simulink model "sininput"  (Simulink 4.00)
settings: Solver=ode45  StartTime=0.0  StopTime=10.0  RelTol=1e-3
settings Model: LastModifiedBy=administrator

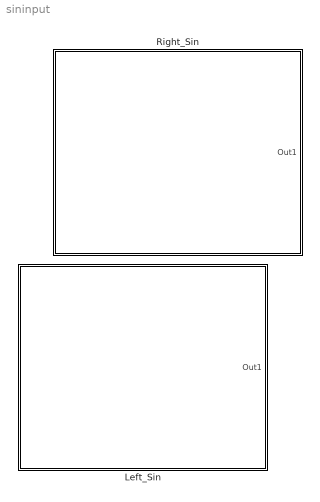
== system sininput ==
  Left_Sin : Subsystem
      settings: RTWFcnNameOpts=Auto  RTWFileNameOpts=Auto
      mask Display: disp('Left_Sin Roadspectrum')
  Right_Sin : Subsystem
      settings: RTWFcnNameOpts=Auto  RTWFileNameOpts=Auto
      mask Display: disp('Right_Sin Roadspectrum')

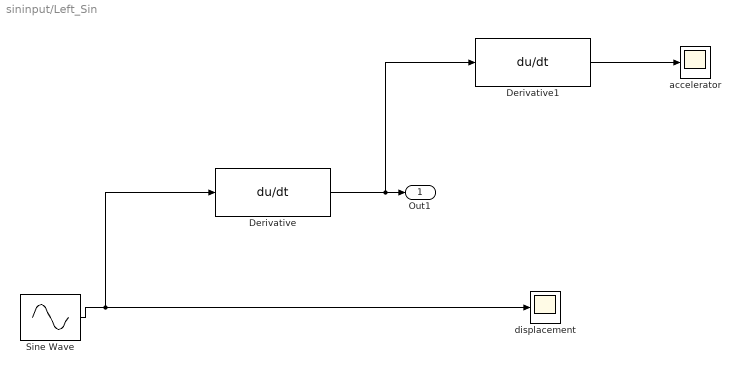
== system sininput/Left_Sin ==
  Derivative : Derivative
  Derivative1 : Derivative
  Sine Wave : Sin  SineType=Time-based  Amplitude=0.015  Bias=0  Frequency=0.5  Phase=0  Samples=10  SampleTime=0  Offset=0
  accelerator : Scope
      settings: TimeRange=auto  YMin=-5  YMax=5  SaveToWorkspace=off  SaveName=ScopeData2  LimitDataPoints=on  MaxDataPoints=5000
  displacement : Scope
      settings: TimeRange=auto  YMin=-5  YMax=5  SaveToWorkspace=off  SaveName=ScopeData  LimitDataPoints=on  MaxDataPoints=5000
  Out1 : Outport  Port=1
  wires:
  Sine Wave/1 -> displacement/1, Derivative/1
  Derivative/1 -> Derivative1/1, Out1/1
  Derivative1/1 -> accelerator/1

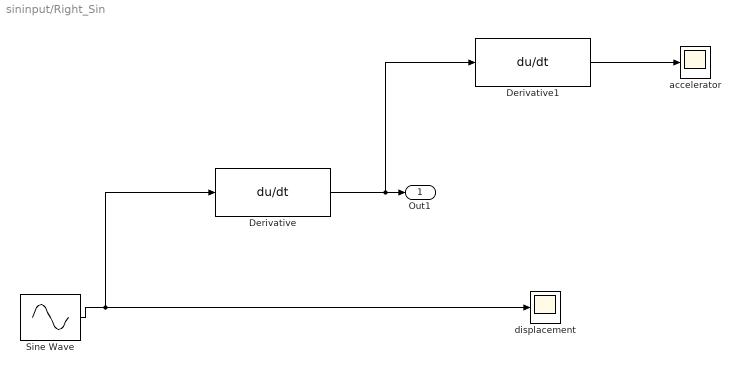
== system sininput/Right_Sin ==
  Derivative : Derivative
  Derivative1 : Derivative
  Sine Wave : Sin  SineType=Time-based  Amplitude=0.015  Bias=0  Frequency=2  Phase=0  Samples=10  SampleTime=0  Offset=0
  accelerator : Scope
      settings: TimeRange=auto  YMin=-5  YMax=5  SaveToWorkspace=off  SaveName=ScopeData2  LimitDataPoints=on  MaxDataPoints=5000
  displacement : Scope
      settings: TimeRange=auto  YMin=-5  YMax=5  SaveToWorkspace=off  SaveName=ScopeData  LimitDataPoints=on  MaxDataPoints=5000
  Out1 : Outport  Port=1
  wires:
  Sine Wave/1 -> displacement/1, Derivative/1
  Derivative/1 -> Derivative1/1, Out1/1
  Derivative1/1 -> accelerator/1
